simulink model "CSTR_model_simulink"  (R2023a)
settings: Solver=ode45  StartTime=0.0  StopTime=30  RelTol=1e-3
settings Model: Creator=owner  LastModifiedBy=Owner

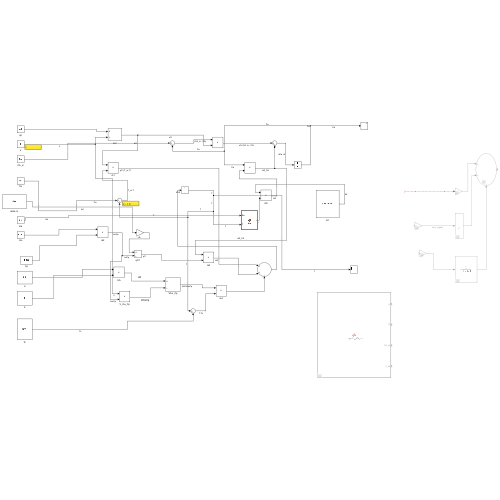
[thumbnail: Simulink's stored preview of the top-level diagram]
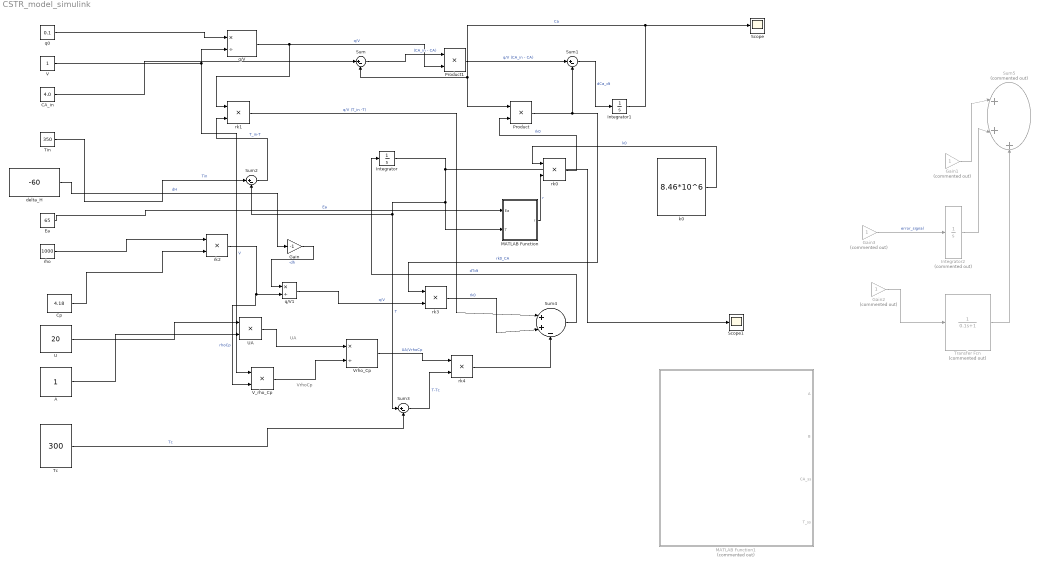
== system CSTR_model_simulink ==
  note: UA
  note: VrhoCp
  A : Constant
  CA_in : Constant  Value=4.0
  Cp : Constant  Value=4.18
  Ea : Constant  Value=65
  Gain : Gain  Gain=-1
  Gain1 : Gain  Commented=on
  Gain2 : Gain  Commented=on
  Gain3 : Gain  Commented=on
  Integrator : Integrator  InitialCondition=350
  Integrator1 : Integrator  InitialCondition=4
  Integrator2 : Integrator  Commented=on
  MATLAB Function : MATLAB Function  TreatAsAtomicUnit=on
  MATLAB Function1 : MATLAB Function  Commented=on  TreatAsAtomicUnit=on
  Product : Product
  Product1 : Product
  Scope : Scope
  Scope1 : Scope
  Sum{,1..3} (4 alike) : Sum  Inputs=|+-
  Sum4 : Sum  Inputs=|++-
  Sum5 : Sum  Commented=on  Inputs=|+++
  Tc : Constant  Value=300
  Tin : Constant  Value=350
  Transfer Fcn : TransferFcn  Commented=on  Denominator=[0.1 1]
  U : Constant  Value=20
  UA : Product
  V : Constant
  V_rho_Cp : Product
  Vrho_Cp : Product  Inputs=*/  RndMeth=Zero  SaturateOnIntegerOverflow=on
  delta_H : Constant  Value=-60
  k0 : Constant  Value=8.46*10^6
  q/V : Product  Inputs=*/  RndMeth=Zero  SaturateOnIntegerOverflow=on
  q/V1 : Product  Inputs=*/  RndMeth=Zero  SaturateOnIntegerOverflow=on
  q0 : Constant  Value=0.1
  rho : Constant  Value=1000
  rk{0..4} (5 alike) : Product
  wires:
  Integrator1/1 -> Product/1, Sum/2, Scope/1  "Ca"
  Sum1/1 -> Integrator1/1  "dCa_dt"
  Integrator/1 -> Scope1/1, Sum3/1, Sum2/2, MATLAB Function/2(T)  "T"
  Sum4/1 -> Integrator/1  "dTdt"
  Ea/1 -> MATLAB Function/1(Ea)  "Ea"
  MATLAB Function/1(r) -> rk0/2  "r"
  k0/1 -> rk0/1  "k0"
  rk0/1 -> Product/2  "rk0"
  CA_in/1 -> Sum/1
  q0/1 -> q/V/1
  V/1 -> q/V/2, V_rho_Cp/1  "V"
  q/V/1 -> rk1/1, Product1/2  "q/V"
  Product1/1 -> Sum1/1  "q/V (CA_in - CA)"
  Sum/1 -> Product1/1  "(CA_in - CA)"
  Product/1 -> rk3/1, Sum1/2  "rk0_CA"
  Tin/1 -> Sum2/1  "Tin"
  Sum2/1 -> rk1/2  "T_in-T"
  rk1/1 -> Sum4/1  "q/V (T_in -T)"
  Cp/1 -> rk2/2
  rho/1 -> rk2/1
  delta_H/1 -> Gain/1  "dH"
  rk2/1 -> V_rho_Cp/2, q/V1/2  "rhoCp"
  q/V1/1 -> rk3/2  "q/V"
  Gain/1 -> q/V1/1  "-dh"
  U/1 -> UA/1
  A/1 -> UA/2
  V_rho_Cp/1 -> Vrho_Cp/2
  UA/1 -> Vrho_Cp/1
  Tc/1 -> Sum3/2  "Tc"
  Vrho_Cp/1 -> rk4/1  "UA/VrhoCp"
  Sum3/1 -> rk4/2  "T-Tc"
  rk4/1 -> Sum4/3
  rk3/1 -> Sum4/2  "rk0"
  Gain3/1 -> Integrator2/1  "error_signal"
  ? -> Gain1/1
  Gain2/1 -> Transfer Fcn/1
  Gain1/1 -> Sum5/1
  Integrator2/1 -> Sum5/2
  Transfer Fcn/1 -> Sum5/3

== matlab function CSTR_model_simulink/MATLAB Function1 ==
  data: A output; B output; CA_ss output; T_ss output
function [A,B,CA_ss,T_ss] = compute_AB_ss()
% Computes steady-state and linearized matrices for non-isothermal CSTR

%% PARAMETERS
V = 1.0;        % Reactor volume [m³]
rho = 1000;     % Density [kg/m³]
Cp = 4.18;      % Heat capacity [kJ/kg·K]
k0 = 8.46e6;    % Pre-exponential factor [1/s]
Ea = 65;        % Activation energy [kJ/mol]
R = 0.008314;   % Gas constant [kJ/mol·K]
deltaH = -60;   % Heat of reaction [kJ/mol]
UA = 20;        % Heat transfer coefficient [kJ/s·K]
CAin = 4.0;     % Feed concentration
Tin = 350;      % Feed temperature
q = 0.1;        % Base flow
Tc = 300;       % Base coolant temperature

%% 1️⃣ Compute steady-state numerically using fsolve
options = optimoptions('fsolve','Display','off');
ss_eq = @(x)[...
    (q/V)*(CAin - x(1)) - k0*exp(-Ea/(R*x(2)))*x(1);   % dCA/dt=0
    (q/V)*(Tin - x(2)) + (-deltaH/(rho*Cp))*k0*exp(-Ea/(R*x(2)))*x(1) ...
      - (UA/(V*rho*Cp))*(x(2)-Tc)                       % dT/dt=0
];
x_guess = [1; 350];  % initial guess [CA;T]
x_ss = fsolve(ss_eq,x_guess,options);

CA_ss = x_ss(1);
T_ss  = x_ss(2);

%% 2️⃣ Compute linearized A matrix at steady state
dx = 1e-6;  % finite difference step
A = zeros(2,2);

for i=1:2
    x_perturb = x_ss;
    x_perturb(i) = x_perturb(i)+dx;
    
    f1p = (q/V)*(CAin - x_perturb(1)) - k0*exp(-Ea/(R*x_perturb(2)))*x_perturb(1);
    f2p = (q/V)*(Tin - x_perturb(2)) + (-deltaH/(rho*Cp))*k0*exp(-Ea/(R*x_perturb(2)))*x_perturb(1) ...
          - (UA/(V*rho*Cp))*(x_perturb(2)-Tc);
    
    fp = [f1p;f2p];
    
    f0 = [(q/V)*(CAin - CA_ss) - k0*exp(-Ea/(R*T_ss))*CA_ss;
          (q/V)*(Tin - T_ss) + (-deltaH/(rho*Cp))*k0*exp(-Ea/(R*T_ss))*CA_ss ...
          - (UA/(V*rho*Cp))*(T_ss-Tc)];
    
    A(:,i) = (fp - f0)/dx;
end

%% 3️⃣ Compute linearized B matrix at steady state
du = 1e-6;
B = zeros(2,2);

for i=1:2
    u_perturb = [q;Tc];
    u_perturb(i) = u_perturb(i)+du;
    
    f1p = (u_perturb(1)/V)*(CAin - CA_ss) - k0*exp(-Ea/(R*T_ss))*CA_ss;
    f2p = (u_perturb(1)/V)*(Tin - T_ss) + (-deltaH/(rho*Cp))*k0*exp(-Ea/(R*T_ss))*CA_ss ...
          - (UA/(V*rho*Cp))*(T_ss - u_perturb(2));
    
    fp = [f1p;f2p];
    
    f0 = [(q/V)*(CAin - CA_ss) - k0*exp(-Ea/(R*T_ss))*CA_ss;
          (q/V)*(Tin - T_ss) + (-deltaH/(rho*Cp))*k0*exp(-Ea/(R*T_ss))*CA_ss ...
          - (UA/(V*rho*Cp))*(T_ss-Tc)];
    
    B(:,i) = (fp - f0)/du;
end

end

== matlab function CSTR_model_simulink/MATLAB Function ==
  data: Ea input; r output; T input
function r = fcn(Ea,T)
%#codegen
R = 0.008314;

r = exp(-Ea /(R*T));
